simulink model "CompleteModel"  (R2018b)
settings: Solver=VariableStepAuto  StartTime=0.0  StopTime=1000  RelTol=1e-3
values from neighbouring files (symbols this model uses):
  A = [-0.322 0.052 0.028 -1.12 0.002;     0 0 1 -0.001 0;     -10.6 0 -2.87 0.46 -0.65;     6.87 0 -0.04 -0.32 -0.02;     0 0 0 0 -7.5]    [A2.m]    (also in model.m = [-0.322 0.052   0.028   -1.12   0.002; prob3sim.m)
  B = [0 0 0 0 7.5]'    [A2.m]    (also in model.m = [0; 0; 0; 0; 7.5]; prob3sim.m)
  C = [eye(4,5)]    [A2.m]    (also in model.m = cat(2, eye(4), zeros(4,1)); prob3sim.m)
  D = [0 0 0 0]'    [A2.m]    (also in prob3sim.m)
  k_dPhi = (2*z_rollDamp*omeg_NatRoll - a_phi1)/(a_phi2)    [A2.m]    (also in prob3sim.m)
  k_iPhi = 0    [A2.m]    (also in prob3sim.m)
  k_iPsi = omeg_NatPsi^2*(V_g/g)    [A2.m]    (also in prob3sim.m)
  k_pPhi = (z_aMax/e_rollMax)*sign(a_phi2)    [A2.m]    (also in prob3sim.m)
  k_pPsi = 2*z_courseDamp*omeg_NatPsi*(V_g/g)    [A2.m]    (also in prob3sim.m)
libraries: simulink_extras x4
settings Model: Creator=Robert  LastModifiedBy=Robert

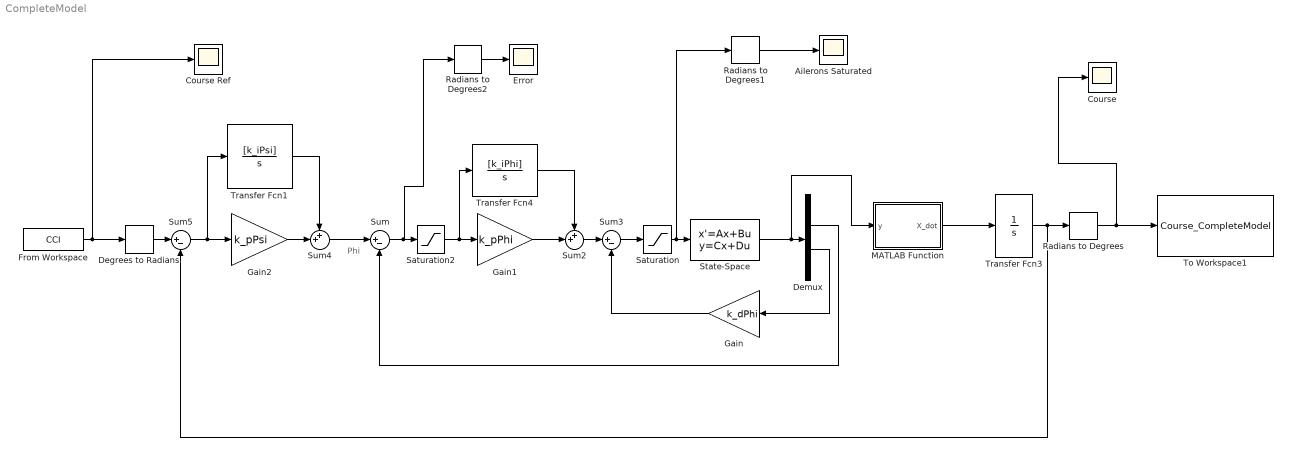
== system CompleteModel ==
  note: Phi
  "Ailerons Saturated " : Scope
  "Course " : Scope
  "Course Ref " : Scope
  Degrees to Radians : simulink_extras/Transformations/Degrees to Radians
  Demux : Demux
  "Error " : Scope
  From Workspace : FromWorkspace  VariableName=CCI  SampleTime=0  Interpolate=off  OutputAfterFinalValue=Holding final value
  Gain : Gain  Gain=k_dPhi
  Gain1 : Gain  Gain=k_pPhi
  Gain2 : Gain  Gain=k_pPsi
  MATLAB Function : MATLAB Function  TreatAsAtomicUnit=on
  Radians to Degrees : simulink_extras/Transformations/Radians to Degrees
  Radians to Degrees1 : simulink_extras/Transformations/Radians to Degrees
  Radians to Degrees2 : simulink_extras/Transformations/Radians to Degrees
  Saturation : Saturate  UpperLimit=30*(pi/180)  LowerLimit=-30*(pi/180)
  Saturation2 : Saturate  UpperLimit=15*(pi/180)  LowerLimit=-15*(pi/180)
  State-Space : StateSpace  A=A  B=B  C=C  D=D  InitialCondition=0
  Sum : Sum  Inputs=|+-
  Sum2 : Sum  Inputs=++|
  Sum3 : Sum  Inputs=|+-
  Sum4 : Sum  Inputs=++|
  Sum5 : Sum  Inputs=|+-
  To Workspace1 : ToWorkspace  VariableName=Course_CompleteModel  SaveFormat=Timeseries  SampleTime=-1
  Transfer Fcn1 : TransferFcn  Numerator=[k_iPsi]  Denominator=[1,0]
  Transfer Fcn3 : TransferFcn  Denominator=[1,0]
  Transfer Fcn4 : TransferFcn  Numerator=[k_iPhi]  Denominator=[1 0]
  wires:
  Transfer Fcn3/1 -> Radians to Degrees/1, Sum5/2
  Sum/1 -> Radians to Degrees2/1, Saturation2/1
  Gain2/1 -> Sum4/2
  Transfer Fcn4/1 -> Sum2/1
  Sum4/1 -> Sum/1
  Gain1/1 -> Sum2/2
  State-Space/1 -> MATLAB Function/1(y), Demux/1
  Demux/2 -> Sum/2
  Sum2/1 -> Sum3/1
  Gain/1 -> Sum3/2
  Demux/3 -> Gain/1
  Sum3/1 -> Saturation/1
  Saturation/1 -> Radians to Degrees1/1, State-Space/1
  MATLAB Function/1(X_dot) -> Transfer Fcn3/1
  From Workspace/1 -> "Course Ref "/1, Degrees to Radians/1
  Degrees to Radians/1 -> Sum5/1
  Radians to Degrees/1 -> "Course "/1, To Workspace1/1
  Sum5/1 -> Transfer Fcn1/1, Gain2/1
  Transfer Fcn1/1 -> Sum4/1
  Radians to Degrees1/1 -> "Ailerons Saturated "/1
  Radians to Degrees2/1 -> "Error "/1
  Saturation2/1 -> Transfer Fcn4/1, Gain1/1

== matlab function CompleteModel/MATLAB Function ==
  data: y input; X_dot output
function X_dot = fcn(y)
    g=9.81;
    V_g=580*(1/3.6);
X_dot = (g/V_g)*tan(y(2)+1.5*(pi/180))*cos(y(1));
